simulink model "Updated_two_trackmodel"  (R2025b)
settings: Solver=ode15s  StartTime=0.0  StopTime=100  MaxStep=0.001  RelTol=1e-3
model workspace (MAT data in the model file):
  A = 1
  Cd = 0.01
  M = 270
  rho = 1.25
libraries: simulink x1
settings Model: PacingRate=0.001000  Creator=vishal bhujbal  LastModifiedBy=vishal bhujbal
settings DebuggingCC: AlgebraicLoopMsg=none

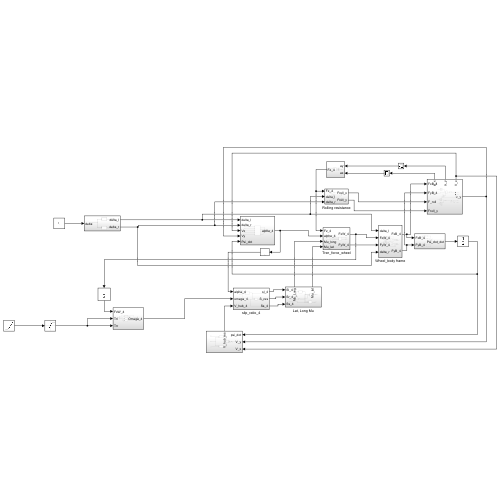
[thumbnail: Simulink's stored preview of the top-level diagram]
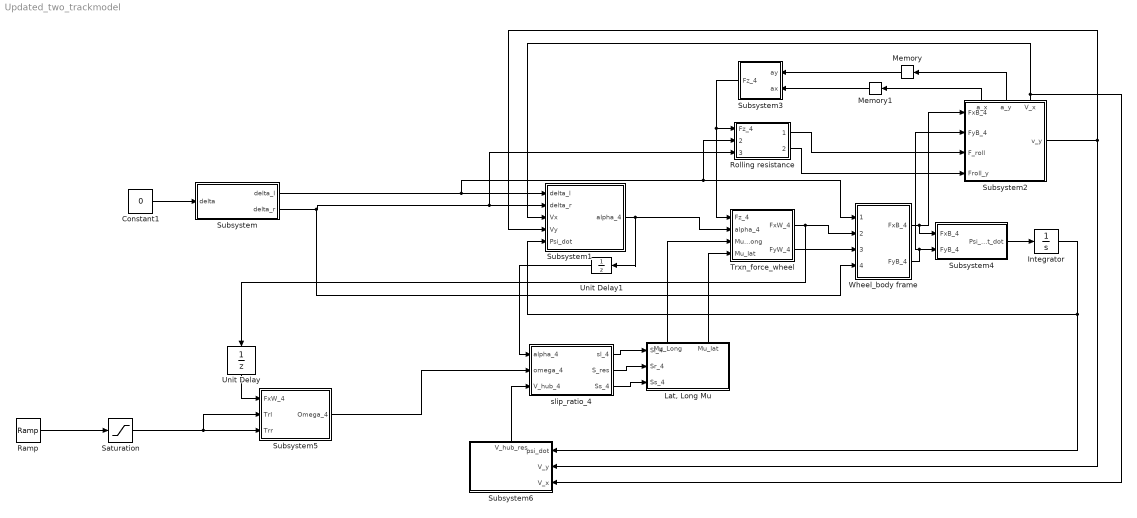
== system Updated_two_trackmodel ==
  Constant1 : Constant  Value=0
  Integrator : Integrator
  "Lat, Long Mu" : Subsystem
      settings: PortSchema="{\"entries\":[{\"content\":{\"sides\":[{\"content\":{\"connectorIds\":[\"In1\",\"In2\",\"In3\"]},\"type\":\"ConnectorPlacement.EquallySpacedRectSide\",\"uuid\":\"075f1f96-cecc-443b-ad9d-28f8dee1470f\"},{\"content\":{\"side\":\"RIGHT\"},\"type\":\"ConnectorPlacement.EquallySpacedRectSide\",\"uuid\":\"85e69d66-dc33-4943-a745-3a3b20a95935\"},{\"content\":{\"connectorIds\":[\"Out1\",\"Out2\"],\"side\":\"TOP\"},\"type\":\"ConnectorPlacement.EquallySpacedRectSide\",\"uuid\":\"b59def5f-074f-4885-80ab-f8315d3dfd66\"}]},\"type\":\"ConnectorPlacement.EquallySpacedConnector\",\"uuid\":\"558734ba-021d-4301-9594-ba1be3f65561\"}],\"packageUris\":[\"http://schema.mathworks.com/mf0/Connector/R2020b\"],\"version\":\"1.0\"}"
  Memory : Memory
  Memory1 : Memory
  Ramp : simulink/Sources/Ramp  slope=9  start=0  InitialOutput=0
  Rolling resistance : Subsystem
  Saturation : Saturate  UpperLimit=29.1  LowerLimit=0
  Subsystem : Subsystem
  Subsystem1 : Subsystem
  Subsystem2 : Subsystem
      settings: PortSchema="{\"entries\":[{\"content\":{\"sides\":[{\"content\":{\"connectorIds\":[\"In1\",\"In2\",\"In3\",\"In4\"]},\"type\":\"ConnectorPlacement.EquallySpacedRectSide\",\"uuid\":\"90e5a5df-8dbe-438b-9274-02268ad6b10b\"},{\"content\":{\"connectorIds\":[\"Out1\"],\"side\":\"RIGHT\"},\"type\":\"ConnectorPlacement.EquallySpacedRectSide\",\"uuid\":\"a74d36ca-41cb-445b-9e7e-3de7340f0617\"},{\"content\":{\"connectorIds\":[\"Out2\",\"Out3\",\"Out4\"],\"side\":\"TOP\"},\"type\":\"ConnectorPlacement.EquallySpacedRectSide\",\"uuid\":\"d4bcddcf-6d65-40cc-9e57-f27c31e929e0\"}]},\"type\":\"ConnectorPlacement.EquallySpacedConnector\",\"uuid\":\"98bc299e-7fcc-49ff-a1d4-bf99aeb78501\"}],\"packageUris\":[\"http://schema.mathworks.com/mf0/Connector/R2020b\"],\"version\":\"1.0\"}"
  Subsystem3 : Subsystem
  Subsystem4 : Subsystem
  Subsystem5 : Subsystem
  Subsystem6 : Subsystem
      settings: PortSchema="{\"entries\":[{\"content\":{\"sides\":[{\"content\":{\"connectorIds\":[\"In1\",\"In2\",\"In3\"]},\"type\":\"ConnectorPlacement.EquallySpacedRectSide\",\"uuid\":\"18c26717-5933-44aa-92c3-7de872a74521\"},{\"content\":{\"side\":\"RIGHT\"},\"type\":\"ConnectorPlacement.EquallySpacedRectSide\",\"uuid\":\"7dd58ecc-b6ac-4a71-b203-3ee3ebed5d1e\"},{\"content\":{\"connectorIds\":[\"Out1\"],\"side\":\"TOP\"},\"type\":\"ConnectorPlacement.EquallySpacedRectSide\",\"uuid\":\"a536145c-5691-43e7-9ef1-fa8170eb65e4\"}]},\"type\":\"ConnectorPlacement.EquallySpacedConnector\",\"uuid\":\"9067e6e1-7c84-4768-9681-1099ff4f2c51\"}],\"packageUris\":[\"http://schema.mathworks.com/mf0/Connector/R2020b\"],\"version\":\"1.0\"}"
  Trxn_force_wheel : Subsystem
  Unit Delay : UnitDelay  SampleTime=-1  HasFrameUpgradeWarning=on
  Unit Delay1 : UnitDelay  SampleTime=-1  HasFrameUpgradeWarning=on
  Wheel_body frame : Subsystem
  slip_ratio_4 : Subsystem
  wires:
  Subsystem/1(delta_l) -> Rolling resistance/2(delta_l), Wheel_body frame/1(delta_l), Subsystem1/1(delta_l)
  Subsystem/2(delta_r) -> Wheel_body frame/4(delta_r), Rolling resistance/3(delta_r), Subsystem1/2(delta_r)
  slip_ratio_4/1(sl_4) -> "Lat, Long Mu"/1(Sl_4)
  slip_ratio_4/2(S_res) -> "Lat, Long Mu"/2(Sr_4)
  slip_ratio_4/3(Ss_4) -> "Lat, Long Mu"/3(Ss_4)
  Subsystem1/1(alpha_4) -> Unit Delay1/1, Trxn_force_wheel/2(alpha_4)
  "Lat, Long Mu"/2(Mu_lat) -> Trxn_force_wheel/4(Mu_lat)
  "Lat, Long Mu"/1(Mu_Long) -> Trxn_force_wheel/3(Mu_long)
  Subsystem3/1(Fz_4) -> Trxn_force_wheel/1(Fz_4), Rolling resistance/1(Fz_4)
  Trxn_force_wheel/1(FxW_4) -> Unit Delay/1, Wheel_body frame/2(FxW_4)
  Trxn_force_wheel/2(FyW_4) -> Wheel_body frame/3(FyW_4)
  Wheel_body frame/1(FxB_4) -> Subsystem2/1(FxB_4), Subsystem4/1(FxB_4)
  Wheel_body frame/2(FyB_4) -> Subsystem2/2(FyB_4), Subsystem4/2(FyB_4)
  Subsystem4/1(Psi_dot_dot) -> Integrator/1
  Integrator/1 -> Subsystem6/1(psi_dot), Subsystem1/5(Psi_dot)
  Saturation/1 -> Subsystem5/2(Trl), Subsystem5/3(Trr)
  Rolling resistance/1(Froll_x) -> Subsystem2/3(F_roll)
  Subsystem2/2(a_x) -> Memory1/1
  Subsystem2/3(a_y) -> Memory/1
  Subsystem2/4(V_x) -> Subsystem1/3(Vx), Subsystem6/3(V_x)
  Subsystem2/1(v_y) -> Subsystem1/4(Vy), Subsystem6/2(V_y)
  Rolling resistance/2(Froll_y) -> Subsystem2/4(Froll_y)
  Subsystem5/1(Omega_4) -> slip_ratio_4/2(omega_4)
  Subsystem6/1(V_hub_res) -> slip_ratio_4/3(V_hub_4)
  Constant1/1 -> Subsystem/1(delta)
  Memory/1 -> Subsystem3/1(ay)
  Memory1/1 -> Subsystem3/2(ax)
  Ramp/1 -> Saturation/1
  Unit Delay/1 -> Subsystem5/1(FxW_4)
  Unit Delay1/1 -> slip_ratio_4/1(alpha_4)

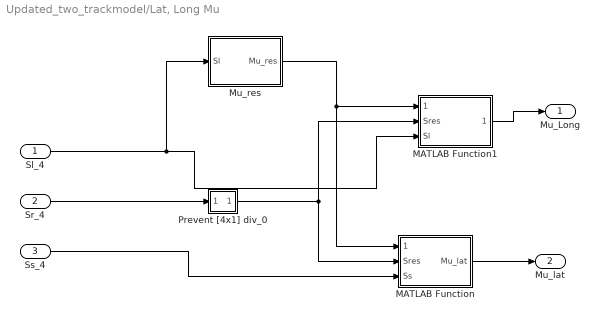
== system Updated_two_trackmodel/Lat, Long Mu ==
  Sl_4 : Inport
  Sr_4 : Inport  Port=2
  Ss_4 : Inport  Port=3
  MATLAB Function : MATLAB Function  TreatAsAtomicUnit=on
  MATLAB Function1 : MATLAB Function  TreatAsAtomicUnit=on
  Mu_res : MATLAB Function  TreatAsAtomicUnit=on
  Prevent [4x1] div_0 : Subsystem
  Mu_Long : Outport
  Mu_lat : Outport  Port=2
  wires:
  Sl_4/1 -> MATLAB Function1/3(Sl), Mu_res/1(Sl)
  Mu_res/1(Mu_res) -> MATLAB Function/1(Mu_res), MATLAB Function1/1(Mu_res)
  Sr_4/1 -> Prevent [4x1] div_0/1(In1)
  Prevent [4x1] div_0/1(Sres) -> MATLAB Function1/2(Sres), MATLAB Function/2(Sres)
  MATLAB Function/1(Mu_lat) -> Mu_lat/1
  Ss_4/1 -> MATLAB Function/3(Ss)
  MATLAB Function1/1(Mu_long) -> Mu_Long/1

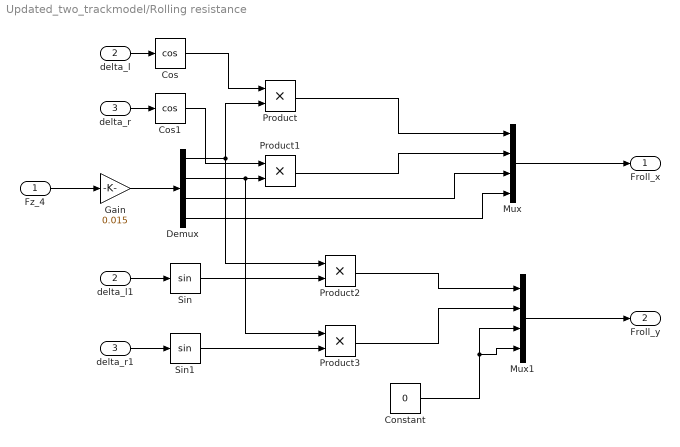
== system Updated_two_trackmodel/Rolling resistance ==
  Fz_4 : Inport
  delta_l : Inport  Port=2
  delta_r : Inport  Port=3
  Constant : Constant  Value=0
  Cos : Trigonometry  Operator=cos
  Cos1 : Trigonometry  Operator=cos
  Demux : Demux
  Gain : Gain  Gain=0.015
  Mux : Mux
  Mux1 : Mux
  Product{,1..3} (4 alike) : Product
  Sin : Trigonometry
  Sin1 : Trigonometry
  delta_l1 : InportShadow  Port=2
  delta_r1 : InportShadow  Port=3
  Froll_x : Outport
  Froll_y : Outport  Port=2
  wires:
  Fz_4/1 -> Gain/1
  Mux/1 -> Froll_x/1
  Demux/1 -> Product2/1, Product/2
  Gain/1 -> Demux/1
  delta_l/1 -> Cos/1
  Cos/1 -> Product/1
  delta_r/1 -> Cos1/1
  Cos1/1 -> Product1/1
  Demux/2 -> Product3/1, Product1/2
  Product/1 -> Mux/1
  Product1/1 -> Mux/2
  Demux/3 -> Mux/3
  Demux/4 -> Mux/4
  delta_l1/1 -> Sin/1
  Sin/1 -> Product2/2
  delta_r1/1 -> Sin1/1
  Sin1/1 -> Product3/2
  Product2/1 -> Mux1/1
  Product3/1 -> Mux1/2
  Constant/1 -> Mux1/4, Mux1/3
  Mux1/1 -> Froll_y/1

== system Updated_two_trackmodel/Subsystem ==
  delta : Inport
  MATLAB Function : MATLAB Function  TreatAsAtomicUnit=on
  MATLAB Function1 : MATLAB Function  TreatAsAtomicUnit=on
  delta_l : Outport
  delta_r : Outport  Port=2
  wires:
  delta/1 -> MATLAB Function1/1(delta), MATLAB Function/1(delta)
  MATLAB Function1/1(delta_r) -> delta_r/1
  MATLAB Function/1(delta_l) -> delta_l/1

== system Updated_two_trackmodel/Subsystem1 ==
  delta_l : Inport
  delta_r : Inport  Port=2
  Vx : Inport  Port=3
  Vy : Inport  Port=4
  Psi_dot : Inport  Port=5
  MATLAB Function : MATLAB Function  TreatAsAtomicUnit=on
  Mux : Mux
  alpha_4 : Outport
  wires:
  MATLAB Function/1(alpha_fl) -> Mux/1
  MATLAB Function/2(alpha_fr) -> Mux/2
  MATLAB Function/3(alpha_rl) -> Mux/3
  MATLAB Function/4(alpha_rr) -> Mux/4
  Mux/1 -> alpha_4/1
  delta_l/1 -> MATLAB Function/1(delta_l)
  delta_r/1 -> MATLAB Function/2(delta_r)
  Vx/1 -> MATLAB Function/3(Vx)
  Vy/1 -> MATLAB Function/4(Vy)
  Psi_dot/1 -> MATLAB Function/5(psi_dot)

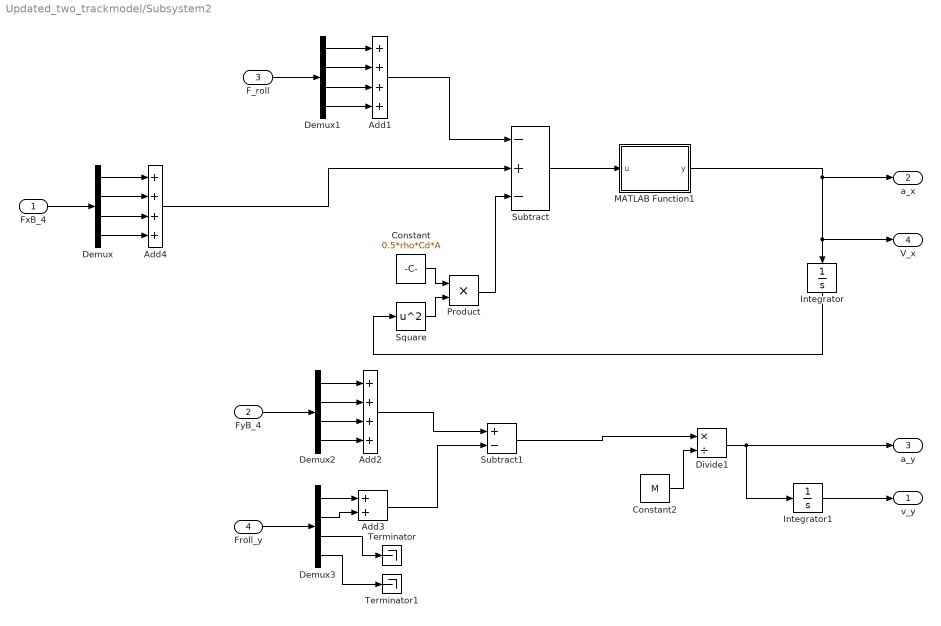
== system Updated_two_trackmodel/Subsystem2 ==
  FxB_4 : Inport
  FyB_4 : Inport  Port=2
  F_roll : Inport  Port=3
  Froll_y : Inport  Port=4
  Add1 : Sum  Inputs=++++
  Add2 : Sum  Inputs=++++
  Add3 : Sum
  Add4 : Sum  Inputs=++++
  Constant : Constant  Value=0.5*rho*Cd*A
  Constant2 : Constant  Value=M
  Demux{,1..3} (4 alike) : Demux
  Divide1 : Product  Inputs=*/
  Integrator : Integrator
  Integrator1 : Integrator
  MATLAB Function1 : MATLAB Function  TreatAsAtomicUnit=on
  Product : Product
  Square : Math  Operator=square
  Subtract : Sum  Inputs=-+-
  Subtract1 : Sum  Inputs=+-
  Terminator : Terminator
  Terminator1 : Terminator
  v_y : Outport
  a_x : Outport  Port=2
  a_y : Outport  Port=3
  V_x : Outport  Port=4
  wires:
  FxB_4/1 -> Demux/1
  F_roll/1 -> Demux1/1
  Demux1/1 -> Add1/1
  Demux1/2 -> Add1/2
  Demux1/3 -> Add1/3
  Demux1/4 -> Add1/4
  Add1/1 -> Subtract/1
  Constant/1 -> Product/1
  Square/1 -> Product/2
  Product/1 -> Subtract/3
  Subtract/1 -> MATLAB Function1/1(u)
  MATLAB Function1/1(y) -> Integrator/1, V_x/1, a_x/1
  FyB_4/1 -> Demux2/1
  Demux2/1 -> Add2/1
  Demux2/2 -> Add2/2
  Demux2/3 -> Add2/3
  Demux2/4 -> Add2/4
  Constant2/1 -> Divide1/2
  Divide1/1 -> Integrator1/1, a_y/1
  Integrator1/1 -> v_y/1
  Add2/1 -> Subtract1/1
  Froll_y/1 -> Demux3/1
  Demux3/1 -> Add3/1
  Demux3/2 -> Add3/2
  Add3/1 -> Subtract1/2
  Demux3/3 -> Terminator/1
  Demux3/4 -> Terminator1/1
  Subtract1/1 -> Divide1/1
  Integrator/1 -> Square/1
  Add4/1 -> Subtract/2
  Demux/1 -> Add4/1
  Demux/2 -> Add4/2
  Demux/3 -> Add4/3
  Demux/4 -> Add4/4

== system Updated_two_trackmodel/Subsystem3 ==
  ay : Inport
  ax : Inport  Port=2
  MATLAB Function : MATLAB Function  TreatAsAtomicUnit=on
  Mux : Mux
  Fz_4 : Outport
  wires:
  MATLAB Function/1(Fzfl) -> Mux/1
  MATLAB Function/2(Fzfr) -> Mux/2
  MATLAB Function/3(Fzrl) -> Mux/3
  MATLAB Function/4(Fzrr) -> Mux/4
  ax/1 -> MATLAB Function/1(ax)
  ay/1 -> MATLAB Function/2(ay)
  Mux/1 -> Fz_4/1

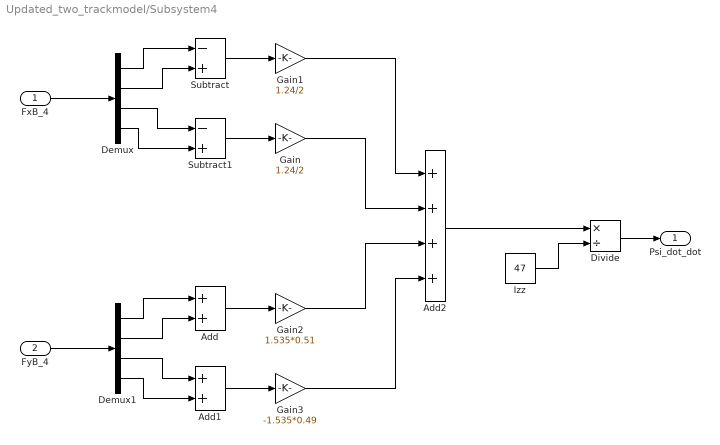
== system Updated_two_trackmodel/Subsystem4 ==
  FxB_4 : Inport
  FyB_4 : Inport  Port=2
  Add : Sum
  Add1 : Sum
  Add2 : Sum  Inputs=++++
  Demux : Demux
  Demux1 : Demux
  Divide : Product  Inputs=*/
  Gain : Gain  Gain=1.24/2
  Gain1 : Gain  Gain=1.24/2
  Gain2 : Gain  Gain=1.535*0.51
  Gain3 : Gain  Gain=-1.535*0.49
  Izz : Constant  Value=47
  Subtract : Sum  Inputs=-+
  Subtract1 : Sum  Inputs=-+
  Psi_dot_dot : Outport
  wires:
  FxB_4/1 -> Demux/1
  Demux/1 -> Subtract/1
  Demux/2 -> Subtract/2
  Demux/3 -> Subtract1/1
  Demux/4 -> Subtract1/2
  Subtract1/1 -> Gain/1
  Subtract/1 -> Gain1/1
  FyB_4/1 -> Demux1/1
  Demux1/1 -> Add/1
  Demux1/2 -> Add/2
  Demux1/3 -> Add1/1
  Demux1/4 -> Add1/2
  Add1/1 -> Gain3/1
  Add/1 -> Gain2/1
  Gain1/1 -> Add2/1
  Gain/1 -> Add2/2
  Gain2/1 -> Add2/3
  Gain3/1 -> Add2/4
  Add2/1 -> Divide/1
  Izz/1 -> Divide/2
  Divide/1 -> Psi_dot_dot/1

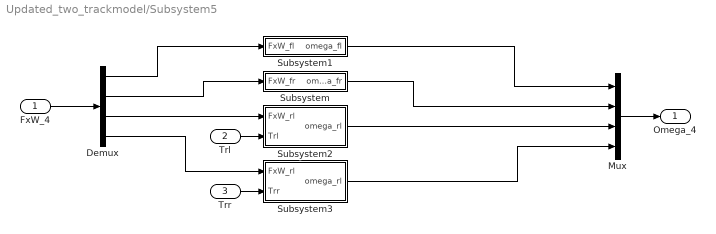
== system Updated_two_trackmodel/Subsystem5 ==
  FxW_4 : Inport
  Trl : Inport  Port=2
  Trr : Inport  Port=3
  Demux : Demux
  Mux : Mux
  Subsystem : Subsystem
  Subsystem1 : Subsystem
  Subsystem2 : Subsystem
  Subsystem3 : Subsystem
  Omega_4 : Outport
  wires:
  FxW_4/1 -> Demux/1
  Demux/2 -> Subsystem/1(FxW_fr)
  Demux/1 -> Subsystem1/1(FxW_fl)
  Demux/3 -> Subsystem2/1(FxW_rl)
  Demux/4 -> Subsystem3/1(FxW_rl)
  Trl/1 -> Subsystem2/2(Trl)
  Trr/1 -> Subsystem3/2(Trr)
  Subsystem1/1(omega_fl) -> Mux/1
  Subsystem/1(omega_fr) -> Mux/2
  Subsystem2/1(omega_rl) -> Mux/3
  Subsystem3/1(omega_rl) -> Mux/4
  Mux/1 -> Omega_4/1

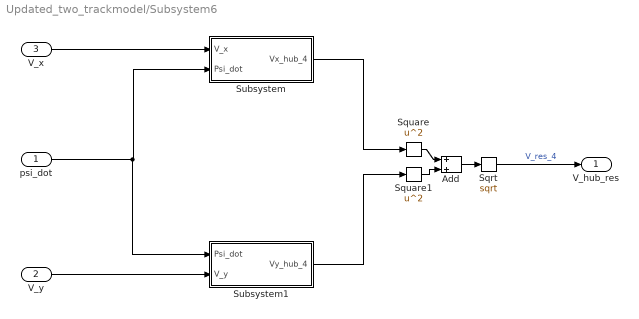
== system Updated_two_trackmodel/Subsystem6 ==
  psi_dot : Inport
  V_y : Inport  Port=2
  V_x : Inport  Port=3
  Add : Sum
  Sqrt : Sqrt
  Square : Math  Operator=square
  Square1 : Math  Operator=square
  Subsystem : Subsystem
  Subsystem1 : Subsystem
  V_hub_res : Outport
  wires:
  V_x/1 -> Subsystem/1(V_x)
  psi_dot/1 -> Subsystem1/1(Psi_dot), Subsystem/2(Psi_dot)
  V_y/1 -> Subsystem1/2(V_y)
  Subsystem/1(Vx_hub_4) -> Square/1
  Subsystem1/1(Vy_hub_4) -> Square1/1
  Square1/1 -> Add/2
  Square/1 -> Add/1
  Add/1 -> Sqrt/1
  Sqrt/1 -> V_hub_res/1  "V_res_4"

== system Updated_two_trackmodel/Trxn_force_wheel ==
  Fz_4 : Inport
  alpha_4 : Inport  Port=2
  Mu_long : Inport  Port=3
  Mu_lat : Inport  Port=4
  MATLAB Function : MATLAB Function  TreatAsAtomicUnit=on
  FxW_4 : Outport
  FyW_4 : Outport  Port=2
  wires:
  MATLAB Function/2(Fyw) -> FyW_4/1
  MATLAB Function/1(Fxw) -> FxW_4/1
  alpha_4/1 -> MATLAB Function/1(alpha_4)
  Mu_lat/1 -> MATLAB Function/2(Mu_lat)
  Mu_long/1 -> MATLAB Function/3(Mu_long)
  Fz_4/1 -> MATLAB Function/4(Fz_4)

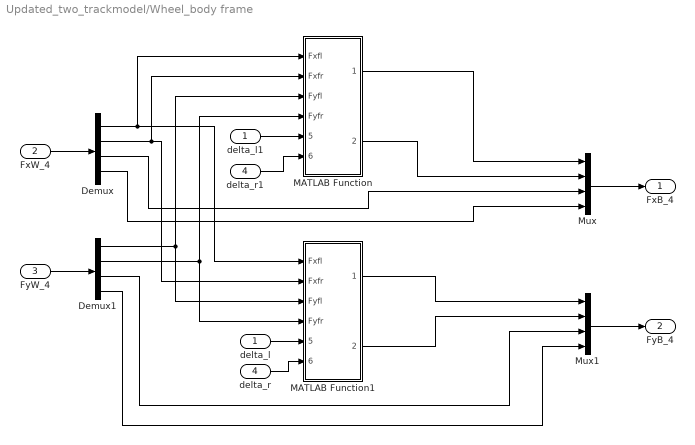
== system Updated_two_trackmodel/Wheel_body frame ==
  delta_l : Inport
  FxW_4 : Inport  Port=2
  FyW_4 : Inport  Port=3
  delta_r : Inport  Port=4
  Demux : Demux
  Demux1 : Demux
  MATLAB Function : MATLAB Function  TreatAsAtomicUnit=on
  MATLAB Function1 : MATLAB Function  TreatAsAtomicUnit=on
  Mux : Mux
  Mux1 : Mux
  delta_l1 : InportShadow
  delta_r1 : InportShadow  Port=4
  FxB_4 : Outport
  FyB_4 : Outport  Port=2
  wires:
  FxW_4/1 -> Demux/1
  Demux/1 -> MATLAB Function1/1(Fxfl), MATLAB Function/1(Fxfl)
  Demux/2 -> MATLAB Function1/2(Fxfr), MATLAB Function/2(Fxfr)
  FyW_4/1 -> Demux1/1
  Demux1/1 -> MATLAB Function1/3(Fyfl), MATLAB Function/3(Fyfl)
  Demux1/2 -> MATLAB Function1/4(Fyfr), MATLAB Function/4(Fyfr)
  delta_l1/1 -> MATLAB Function/5(delta_l)
  delta_r1/1 -> MATLAB Function/6(delta_r)
  delta_l/1 -> MATLAB Function1/5(delta_l)
  delta_r/1 -> MATLAB Function1/6(delta_r)
  MATLAB Function/1(FxflB) -> Mux/1
  MATLAB Function/2(FxfrB) -> Mux/2
  Demux/3 -> Mux/3
  Demux/4 -> Mux/4
  Demux1/3 -> Mux1/3
  Demux1/4 -> Mux1/4
  MATLAB Function1/1(FyflB) -> Mux1/1
  MATLAB Function1/2(FyfrB) -> Mux1/2
  Mux/1 -> FxB_4/1
  Mux1/1 -> FyB_4/1

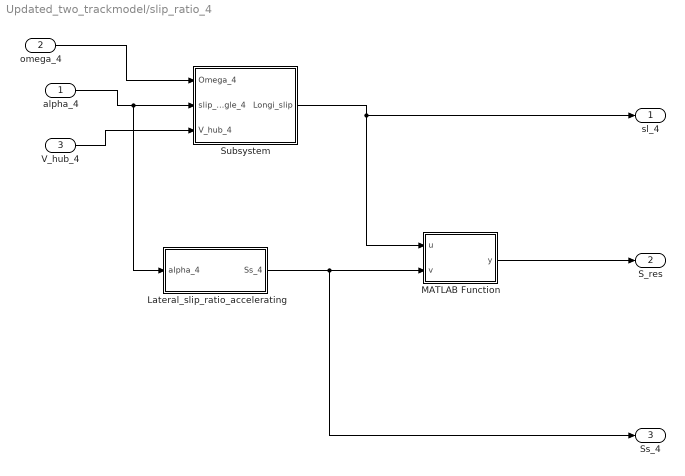
== system Updated_two_trackmodel/slip_ratio_4 ==
  alpha_4 : Inport
  omega_4 : Inport  Port=2
  V_hub_4 : Inport  Port=3
  Lateral_slip_ratio_accelerating : Subsystem
  MATLAB Function : MATLAB Function  TreatAsAtomicUnit=on
  Subsystem : Subsystem
  sl_4 : Outport
  S_res : Outport  Port=2
  Ss_4 : Outport  Port=3
  wires:
  omega_4/1 -> Subsystem/1(Omega_4)
  V_hub_4/1 -> Subsystem/3(V_hub_4)
  alpha_4/1 -> Lateral_slip_ratio_accelerating/1(alpha_4), Subsystem/2(slip_angle_4)
  Subsystem/1(Longi_slip) -> MATLAB Function/1(u), sl_4/1
  MATLAB Function/1(y) -> S_res/1
  Lateral_slip_ratio_accelerating/1(Ss_4) -> MATLAB Function/2(v), Ss_4/1

== system Updated_two_trackmodel/Lat, Long Mu/Prevent [4x1] div_0 ==
  In1 : Inport
  Demux : Demux
  MATLAB Function : MATLAB Function  TreatAsAtomicUnit=on
  MATLAB Function1 : MATLAB Function  TreatAsAtomicUnit=on
  MATLAB Function2 : MATLAB Function  TreatAsAtomicUnit=on
  MATLAB Function3 : MATLAB Function  TreatAsAtomicUnit=on
  Mux : Mux
  Sres : Outport
  wires:
  In1/1 -> Demux/1
  Demux/1 -> MATLAB Function/1(u)
  Demux/4 -> MATLAB Function3/1(u)
  Demux/3 -> MATLAB Function2/1(u)
  Demux/2 -> MATLAB Function1/1(u)
  MATLAB Function/1(y) -> Mux/1
  MATLAB Function1/1(y) -> Mux/2
  MATLAB Function2/1(y) -> Mux/3
  MATLAB Function3/1(y) -> Mux/4
  Mux/1 -> Sres/1

== system Updated_two_trackmodel/Subsystem5/Subsystem ==
  FxW_fr : Inport
  Add1 : Sum
  Divide1 : Product  Inputs=/*
  Gain2 : Gain  Gain=-0.228
  Gain3 : Gain  Gain=-0.01
  Integrator1 : Integrator
  Iw1 : Constant  Value=0.65
  omega_fr : Outport
  wires:
  Gain3/1 -> Add1/1
  FxW_fr/1 -> Gain2/1
  Integrator1/1 -> omega_fr/1, Gain3/1
  Iw1/1 -> Divide1/1
  Add1/1 -> Divide1/2
  Gain2/1 -> Add1/2
  Divide1/1 -> Integrator1/1  "omega_dot"

== system Updated_two_trackmodel/Subsystem5/Subsystem1 ==
  FxW_fl : Inport
  Add1 : Sum
  Divide1 : Product  Inputs=/*
  Gain2 : Gain  Gain=-0.228
  Gain3 : Gain  Gain=-0.01
  Integrator1 : Integrator
  Iw1 : Constant  Value=0.65
  omega_fl : Outport
  wires:
  Divide1/1 -> Integrator1/1  "omega_dot"
  Gain2/1 -> Add1/2
  Add1/1 -> Divide1/2
  Iw1/1 -> Divide1/1
  Integrator1/1 -> Gain3/1, omega_fl/1
  FxW_fl/1 -> Gain2/1
  Gain3/1 -> Add1/1

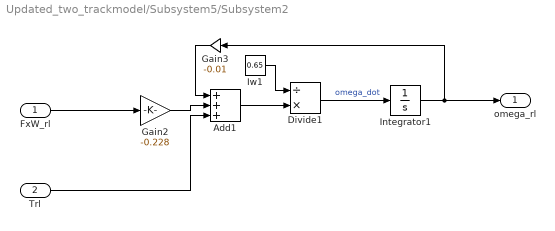
== system Updated_two_trackmodel/Subsystem5/Subsystem2 ==
  FxW_rl : Inport
  Trl : Inport  Port=2
  Add1 : Sum  Inputs=+++
  Divide1 : Product  Inputs=/*
  Gain2 : Gain  Gain=-0.228
  Gain3 : Gain  Gain=-0.01
  Integrator1 : Integrator
  Iw1 : Constant  Value=0.65
  omega_rl : Outport
  wires:
  Divide1/1 -> Integrator1/1  "omega_dot"
  Gain2/1 -> Add1/2
  Add1/1 -> Divide1/2
  Iw1/1 -> Divide1/1
  Integrator1/1 -> Gain3/1, omega_rl/1
  FxW_rl/1 -> Gain2/1
  Gain3/1 -> Add1/1
  Trl/1 -> Add1/3

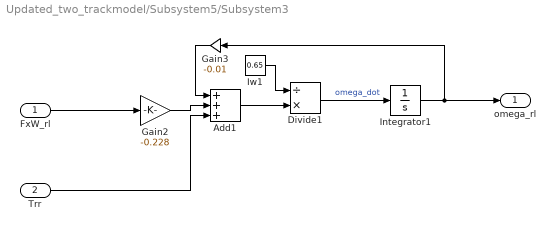
== system Updated_two_trackmodel/Subsystem5/Subsystem3 ==
  FxW_rl : Inport
  Trr : Inport  Port=2
  Add1 : Sum  Inputs=+++
  Divide1 : Product  Inputs=/*
  Gain2 : Gain  Gain=-0.228
  Gain3 : Gain  Gain=-0.01
  Integrator1 : Integrator
  Iw1 : Constant  Value=0.65
  omega_rl : Outport
  wires:
  Trr/1 -> Add1/3
  Gain3/1 -> Add1/1
  FxW_rl/1 -> Gain2/1
  Integrator1/1 -> omega_rl/1, Gain3/1
  Iw1/1 -> Divide1/1
  Add1/1 -> Divide1/2
  Gain2/1 -> Add1/2
  Divide1/1 -> Integrator1/1  "omega_dot"

== system Updated_two_trackmodel/Subsystem6/Subsystem ==
  V_x : Inport
  Psi_dot : Inport  Port=2
  MATLAB Function : MATLAB Function  TreatAsAtomicUnit=on
  Mux : Mux
  Vx_hub_4 : Outport
  wires:
  Psi_dot/1 -> MATLAB Function/2(Psi_dot)
  V_x/1 -> MATLAB Function/1(Vx_vehicle)
  MATLAB Function/1(Vxwfl) -> Mux/1
  MATLAB Function/2(Vxwfr) -> Mux/2
  MATLAB Function/3(Vxwrl) -> Mux/3
  MATLAB Function/4(Vxwrr) -> Mux/4
  Mux/1 -> Vx_hub_4/1

== system Updated_two_trackmodel/Subsystem6/Subsystem1 ==
  Psi_dot : Inport
  V_y : Inport  Port=2
  MATLAB Function : MATLAB Function  TreatAsAtomicUnit=on
  Mux : Mux
  Vy_hub_4 : Outport
  wires:
  Mux/1 -> Vy_hub_4/1
  MATLAB Function/4(Vywrr) -> Mux/4
  MATLAB Function/3(Vywrl) -> Mux/3
  MATLAB Function/2(Vywfr) -> Mux/2
  MATLAB Function/1(Vywfl) -> Mux/1
  V_y/1 -> MATLAB Function/1(Vy_vehicle)
  Psi_dot/1 -> MATLAB Function/2(Psi_dot)

== system Updated_two_trackmodel/slip_ratio_4/Lateral_slip_ratio_accelerating ==
  alpha_4 : Inport
  MATLAB Function : MATLAB Function  TreatAsAtomicUnit=on
  Ss_4 : Outport
  wires:
  alpha_4/1 -> MATLAB Function/1(alpha_4)
  MATLAB Function/1(Ss_4) -> Ss_4/1

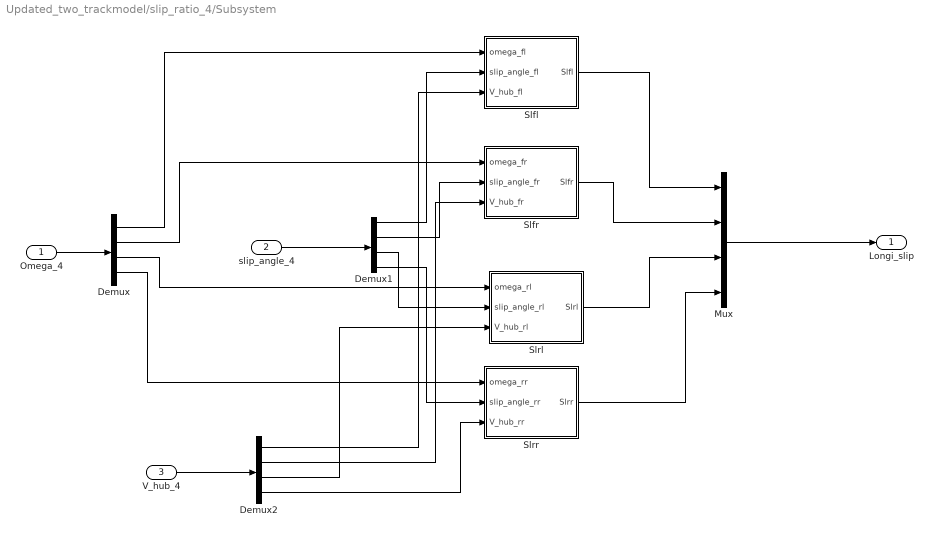
== system Updated_two_trackmodel/slip_ratio_4/Subsystem ==
  Omega_4 : Inport
  slip_angle_4 : Inport  Port=2
  V_hub_4 : Inport  Port=3
  Demux : Demux
  Demux1 : Demux
  Demux2 : Demux
  Mux : Mux
  Slfl : MATLAB Function  TreatAsAtomicUnit=on
  Slfr : MATLAB Function  TreatAsAtomicUnit=on
  Slrl : MATLAB Function  TreatAsAtomicUnit=on
  Slrr : MATLAB Function  TreatAsAtomicUnit=on
  Longi_slip : Outport
  wires:
  Omega_4/1 -> Demux/1
  V_hub_4/1 -> Demux2/1
  slip_angle_4/1 -> Demux1/1
  Demux1/1 -> Slfl/2(slip_angle_fl)
  Demux1/2 -> Slfr/2(slip_angle_fr)
  Demux1/3 -> Slrl/2(slip_angle_rl)
  Demux1/4 -> Slrr/2(slip_angle_rr)
  Demux/1 -> Slfl/1(omega_fl)
  Demux/2 -> Slfr/1(omega_fr)
  Demux/3 -> Slrl/1(omega_rl)
  Demux/4 -> Slrr/1(omega_rr)
  Demux2/1 -> Slfl/3(V_hub_fl)
  Demux2/2 -> Slfr/3(V_hub_fr)
  Demux2/3 -> Slrl/3(V_hub_rl)
  Demux2/4 -> Slrr/3(V_hub_rr)
  Mux/1 -> Longi_slip/1
  Slfl/1(Slfl) -> Mux/1
  Slfr/1(Slfr) -> Mux/2
  Slrl/1(Slrl) -> Mux/3
  Slrr/1(Slrr) -> Mux/4

== matlab function Updated_two_trackmodel/Wheel_body frame/MATLAB Function1 ==
  data: Fxfl input; Fxfr input; FyflB output; Fyfl input; Fyfr input; delta_l input; delta_r input; FyfrB output
function [FyflB,FyfrB] = fcn(Fxfl,Fxfr,Fyfl,Fyfr,delta_l,delta_r)

FyflB = Fxfl*sin(delta_l) + Fyfl*cos(delta_l);
FyfrB = Fxfr*sin(delta_r) + Fyfr*cos(delta_r);

== matlab function Updated_two_trackmodel/Subsystem6/Subsystem/MATLAB Function ==
  data: Vx_vehicle input; Vxwfl output; Psi_dot input; Vxwfr output; Vxwrl output; Vxwrr output
function [Vxwfl,Vxwfr,Vxwrl,Vxwrr] = fcn(Vx_vehicle,Psi_dot)

Rw = 0.228;
tf = 1.24;
tr = 1.24;
Lf = 1.535*0.51;
Lr = 1.535*0.49;

Vxwfl = Vx_vehicle - Psi_dot.*Rw.*sind(tf/(2.*Lf));
Vxwfr = Vx_vehicle + Psi_dot.*Rw.*sind(tf/(2.*Lf));
Vxwrl = Vx_vehicle - Psi_dot.*Rw.*sind(tr/(2.*Lr));
Vxwrr = Vx_vehicle + Psi_dot.*Rw.*sind(tr/(2.*Lr));

== matlab function Updated_two_trackmodel/Subsystem6/Subsystem1/MATLAB Function ==
  data: Vy_vehicle input; Vywfl output; Psi_dot input; Vywfr output; Vywrl output; Vywrr output
function [Vywfl,Vywfr,Vywrl,Vywrr] = fcn(Vy_vehicle,Psi_dot)

Rw = 0.228;
tf = 1.24;
tr = 1.24;
Lf = 1.535*0.51;
Lr = 1.535*0.49;

Vywfl = Vy_vehicle + Psi_dot.*Rw.*cosd(tf/(2.*Lf));
Vywfr = Vy_vehicle + Psi_dot.*Rw.*cosd(tf/(2.*Lf));
Vywrl = Vy_vehicle - Psi_dot.*Rw.*cosd(tr/(2.*Lr));
Vywrr = Vy_vehicle - Psi_dot.*Rw.*cosd(tr/(2.*Lr));

== matlab function Updated_two_trackmodel/slip_ratio_4/Subsystem/Slfl ==
  data: omega_fl input; Slfl output; slip_angle_fl input; V_hub_fl input
function Slfl = fcn(omega_fl,slip_angle_fl,V_hub_fl)
Rw = 0.228;
% numerator
num = omega_fl * Rw * cos(slip_angle_fl) - V_hub_fl;

% raw denominator
den_raw = max(V_hub_fl, omega_fl * Rw * cos(slip_angle_fl));

% create safe denominator:
% - keep the sign
% - avoid zero
% - smooth for solver
den = den_raw+0.00001 ;

% if the raw denominator is exactly zero → choose a tiny positive number
if den_raw == 0
    den = 0.0001;
end

% slip ratio
Slfl = num / den;

== matlab function Updated_two_trackmodel/Subsystem/MATLAB Function1 ==
  data: delta input; delta_r output
function delta_r = fcn(delta)
tf = 1.24;
L = 1.535;
delta_r = atan(L/(L.*cot(delta)+tf/2));

== matlab function Updated_two_trackmodel/slip_ratio_4/Subsystem/Slrl ==
  data: omega_rl input; Slrl output; slip_angle_rl input; V_hub_rl input
function Slrl = fcn(omega_rl,slip_angle_rl,V_hub_rl)
Rw = 0.228;
% numerator
num = omega_rl * Rw * cos(slip_angle_rl) - V_hub_rl;

% raw denominator
den_raw = max(V_hub_rl, omega_rl * Rw * cos(slip_angle_rl));

% create safe denominator:
% - keep the sign
% - avoid zero
% - smooth for solver
den = den_raw+0.00001;

% if the raw denominator is exactly zero → choose a tiny positive number
if den_raw == 0
    den = 0.0001;
end

% slip ratio
Slrl = num / den;

== matlab function Updated_two_trackmodel/slip_ratio_4/Subsystem/Slrr ==
  data: omega_rr input; Slrr output; slip_angle_rr input; V_hub_rr input
function Slrr = fcn(omega_rr, slip_angle_rr, V_hub_rr)
Rw = 0.228;
% numerator
num = omega_rr * Rw * cos(slip_angle_rr) - V_hub_rr;

% raw denominator
den_raw = max(V_hub_rr, omega_rr * Rw * cos(slip_angle_rr));

% create safe denominator:
% - keep the sign
% - avoid zero
% - smooth for solver
den = den_raw +0.00001;

% if the raw denominator is exactly zero → choose a tiny positive number
if den_raw == 0
    den = 0.0001;
end

% slip ratio
Slrr = num / den;

== matlab function Updated_two_trackmodel/Lat, Long Mu/Prevent [4x1] div_0/MATLAB Function1 ==
  data: u input; y output
function y = preventZero(u)
% Prevent ONLY zero, allow negative and positive values

eps_val = 1e-3;          % small positive value

y = u;                   % pass input directly
y(u == 0) = eps_val;     % replace only zero values

end

== matlab function Updated_two_trackmodel/Lat, Long Mu/Prevent [4x1] div_0/MATLAB Function2 ==
  data: u input; y output
function y = preventZero(u)
% Prevent ONLY zero, allow negative and positive values

eps_val = 1e-3;          % small positive value

y = u;                   % pass input directly
y(u == 0) = eps_val;     % replace only zero values

end

== matlab function Updated_two_trackmodel/slip_ratio_4/Lateral_slip_ratio_accelerating/MATLAB Function ==
  data: alpha_4 input; Ss_4 output
function Ss_4 = fcn(alpha_4)

Ss_4 = tan(alpha_4)+0.00001;

== matlab function Updated_two_trackmodel/Lat, Long Mu/Prevent [4x1] div_0/MATLAB Function3 ==
  data: u input; y output
function y = preventZero(u)
% Prevent ONLY zero, allow negative and positive values

eps_val = 1e-3;          % small positive value

y = u;                   % pass input directly
y(u == 0) = eps_val;     % replace only zero values

end

== matlab function Updated_two_trackmodel/Lat, Long Mu/MATLAB Function ==
  data: Mu_res input; Mu_lat output; Sres input; Ss input
function Mu_lat = fcn(Mu_res,Sres,Ss)

Mu_lat = Mu_res.*(Ss./Sres);

== matlab function Updated_two_trackmodel/Lat, Long Mu/MATLAB Function1 ==
  data: Mu_res input; Mu_long output; Sres input; Sl input
function Mu_long = fcn(Mu_res,Sres,Sl)

Mu_long = Mu_res.*(Sl./Sres);

== matlab function Updated_two_trackmodel/Subsystem2/MATLAB Function1 ==
  data: u input; y output
function y = fcn(u)

y = u/270;

== matlab function Updated_two_trackmodel/Subsystem/MATLAB Function ==
  data: delta input; delta_l output
function delta_l = fcn(delta)
tf = 1.24;
L = 1.535;
delta_l = atan(L/(L.*cot(delta)-tf/2));

== matlab function Updated_two_trackmodel/slip_ratio_4/MATLAB Function ==
  data: u input; y output; v input
function y = fcn(u,v)

y = sqrt(u.^2+v.^2);

== matlab function Updated_two_trackmodel/Subsystem1/MATLAB Function ==
  data: delta_l input; delta_r input; alpha_fl output; Vx input; Vy input; psi_dot input; alpha_fr output; alpha_rl output; alpha_rr output
function [alpha_fl,alpha_fr,alpha_rl,alpha_rr] = fcn(delta_l,delta_r,Vx,Vy,psi_dot)
Lf = 1.535*0.51;
tf = 1.24;
Lr = 1.535*0.49;
tr = 1.24;

alpha_fl = delta_l - atan((Vy+psi_dot.*Lf)./(Vx-psi_dot*tf/2))+0.0001;
alpha_fr = delta_r - atan((Vy+psi_dot.*Lf)./(Vx+psi_dot*tf/2))+0.0001;
alpha_rl = -atan((Vy-psi_dot.*Lr)./(Vx-psi_dot*tr/2))+0.0001;
alpha_rr = -atan((Vy-psi_dot.*Lr)./(Vx+psi_dot*tr/2))+0.0001;

== matlab function Updated_two_trackmodel/slip_ratio_4/Subsystem/Slfr ==
  data: omega_fr input; Slfr output; slip_angle_fr input; V_hub_fr input
function Slfr = fcn(omega_fr,slip_angle_fr,V_hub_fr)
Rw = 0.228;
% numerator
num = omega_fr * Rw * cos(slip_angle_fr) - V_hub_fr;

% raw denominator
den_raw = max(V_hub_fr, omega_fr * Rw * cos(slip_angle_fr));

% create safe denominator:
% - keep the sign
% - avoid zero
% - smooth for solver
den = den_raw+0.00001 ;

% if the raw denominator is exactly zero → choose a tiny positive number
if den_raw == 0
    den = 0.0001;
end

% slip ratio
Slfr = num / den;

== matlab function Updated_two_trackmodel/Lat, Long Mu/Prevent [4x1] div_0/MATLAB Function ==
  data: u input; y output
function y = preventZero(u)
% Prevent ONLY zero, allow negative and positive values

eps_val = 1e-3;          % small positive value

y = u;                   % pass input directly
y(u == 0) = eps_val;     % replace only zero values

end

== matlab function Updated_two_trackmodel/Lat, Long Mu/Mu_res ==
  data: Sl input; Mu_res output
function Mu_res = fcn(Sl)
C1 = 1.2801;
C2 = 23.99;
C3 = 0.52;

Mu_res = C1*(1-exp(-C2.*abs(Sl)))-C3*abs(Sl);

== matlab function Updated_two_trackmodel/Subsystem3/MATLAB Function ==
  data: ax input; Fzfl output; ay input; Fzfr output; Fzrl output; Fzrr output
function [Fzfl,Fzfr,Fzrl,Fzrr] = fcn(ax,ay)
M = 270;
Hcg = 0.25;
L = 1.535;
tr = 1.24;
Fzfl = M*9.81/4 - M*ax*Hcg/(2*L) - M*ay*Hcg/tr;
Fzfr = M*9.81/4 - M*ax*Hcg/(2*L) + M*ay*Hcg/tr;
Fzrl = M*9.81/4 + M*ax*Hcg/(2*L) - M*ay*Hcg/tr;
Fzrr = M*9.81/4 + M*ax*Hcg/(2*L) + M*ay*Hcg/tr;

== matlab function Updated_two_trackmodel/Trxn_force_wheel/MATLAB Function ==
  data: alpha_4 input; Fxw output; Mu_lat input; Mu_long input; Fz_4 input; Fyw output
function [Fxw,Fyw] = fcn(alpha_4,Mu_lat,Mu_long,Fz_4)

Fxw = Mu_long.*Fz_4.*cos(alpha_4) + Mu_lat.*Fz_4.*sin(alpha_4);

Fyw = Mu_lat.*Fz_4.*cos(alpha_4) - Mu_long.*Fz_4.*sin(alpha_4);

== matlab function Updated_two_trackmodel/Wheel_body frame/MATLAB Function ==
  data: Fxfl input; Fxfr input; FxflB output; Fyfl input; Fyfr input; delta_l input; delta_r input; FxfrB output
function [FxflB,FxfrB] = fcn(Fxfl,Fxfr,Fyfl,Fyfr,delta_l,delta_r)

FxflB = Fxfl*cos(delta_l) - Fyfl*sin(delta_l);
FxfrB = Fxfr*cos(delta_r) - Fyfr*sin(delta_r);
